simulink model "Freq_SimpleC_mex_new"  (R2020a)
settings: Solver=VariableStepAuto  StartTime=0.0  StopTime=50  FixedStep=0.02  MaxStep=1e-3  RelTol=1e-3
InitFcn:
  | M = 4; D = 1.5/100; Rp = 0.05; Tg = 0.2; Ki = 1.8;
libraries: commchan3 x1
settings Model: Creator=Niranjan.Bhujel  LastModifiedBy=astha.rai

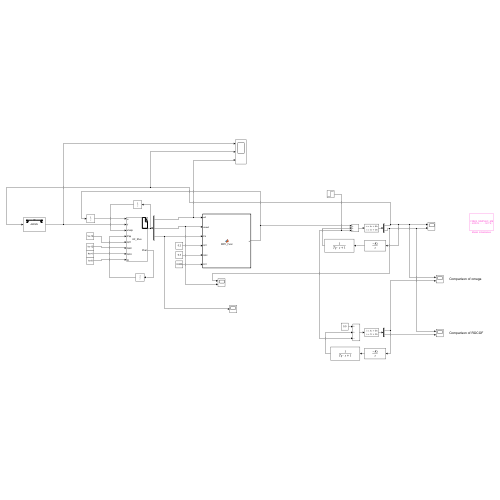
[thumbnail: Simulink's stored preview of the top-level diagram]
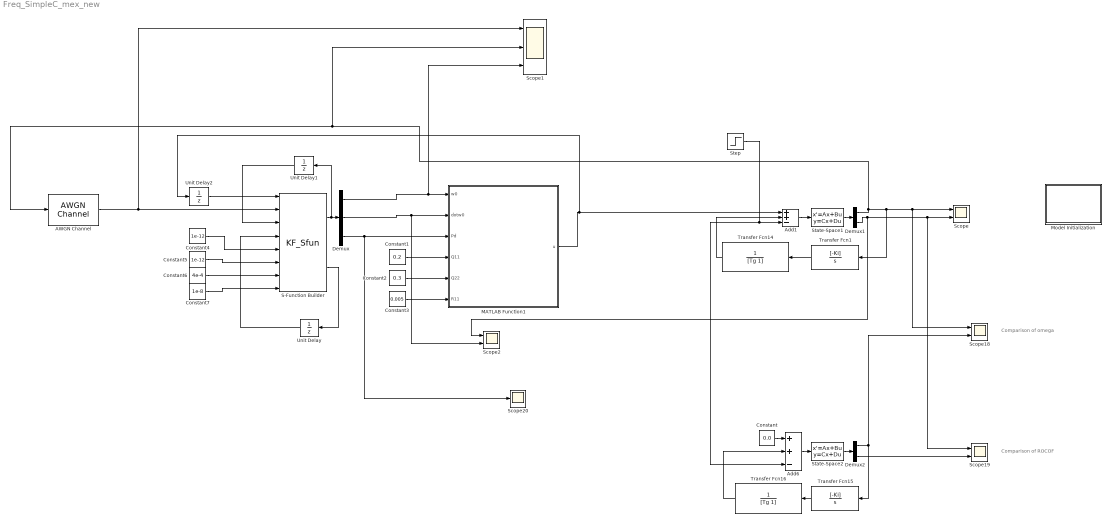
== system Freq_SimpleC_mex_new ==
  note: Comparison of omega
  note: Comparison of ROCOF
  AWGN Channel : commchan3/AWGN Channel  InputProcessing=Columns as channels (frame based)  seed=67  noiseMode=Variance from mask  EbNodB=10  EsNodB=10  SNRdB=10  bitsPerSym=1  Ps=1  Tsym=1  variance=1e-8
  Add1 : Sum  Inputs=++-
  Add6 : Sum  Inputs=++-
  Constant : Constant  Value=0.0
  Constant1 : Constant  Value=0.2
  Constant2 : Constant  Value=0.3
  Constant3 : Constant  Value=0.005
  Constant4 : Constant  Value=1e-12
  Constant5 : Constant  Value=1e-12
  Constant6 : Constant  Value=4e-4
  Constant7 : Constant  Value=1e-8
  Demux : Demux  Outputs=3
  Demux1 : Demux  Outputs=2
  Demux2 : Demux  Outputs=2
  MATLAB Function1 : MATLAB Function  TreatAsAtomicUnit=on  SystemSampleTime=0.02
      settings: MinAlgLoopOccurrences=on
  Model Initialization : Subsystem  mask(Model Functions){InitFcnX=M = 4; D = 1.5/100; Rp = 0.05; Tg = 0.2; Ki = 1.8;, prel=off, posl=off, inif=on, strf=off}
      mask prompts: InitFcnX "Initialisation"; prel "Preload Function"; posl "PostLoad Function"; inif "InitFcn"; strf "StartFcn"
      mask init:
      | currentBlock = gcb;
      | root = bdroot(currentBlock);
      | 
      | if ~strcmp(get_param(root,'BlockDiagramType'),'library')
      |     if prel==1
      |         set_param(root, 'PreLoadFcn', InitFcnX);
      |     else
      |         set_param(root, 'PreLoadFcn', '');
      |     end
      |     if inif==1
      |         set_param(root, 'InitFcn', InitFcnX);
      |     else
      |         set_param(root, 'InitFcn', '');
      |     end
      |     if strf==1
      |         set_param(root, 'StartFcn', InitFcnX);
      |     else
      |         set_param(root, 'StartFcn', '');
      |     end
      |     if posl==1
      |         set_param(root, 'PostLoadFcn', InitFcnX);
      |     else
      |         set_param(root, 'PostLoadFcn', '');
      |     end
      | end
      | 
      | pos = get_param(currentBlock, 'Position');
      | width = pos(3) - pos(1); height = pos(4) - pos(2);
      | txt = [ upper(root) '\n' '- InitFcn. . . . . '  get_param(root, 'InitFcn') ];
      settings: CopyFcn=set_param(gcb,'LinkStatus','inactive')
      mask Display: text(5, height*0.5, txt, 'horizontalAlignment', 'left', 'verticalAlignment', 'middle') ;
  S-Function Builder : S-Function  InitFcn=try, set_param(gcb,'FunctionName','KF_Sfun'), end  FunctionName=KF_Sfun  SFunctionModules=KF_Sfun_wrapper EKF_Func EKF_Func_Call  SFunctionDeploymentMode=off  EnableBusSupport=off  mask(S-Function Builder){}
      mask help: Simulink:masks:SFunctionBuilder_MD
      mask init:
      | val = [[.9  0.75 0.75 1 1 .9 .9 1]',[1 1 0.75 0.75 .9 .9 1 .9]'];try , sys = get_param(gcb,'SfunBuilderFcnName');if isempty(sys), sys = get_param(gcb,'FunctionName'); end,catch, sys = get_param(gcb,'FunctionName'); end
      settings: CopyFcn=set_param(gcbh,'LinkStatus','none')  PreSaveFcn=try, set_param(gcb,'FunctionName','KF_Sfun'), end  OpenFcn=sfunctionwizard(gcbh)
      mask Display:
      | plot(val(:,1),val(:,2))
      | disp(sys)
      | port_label('input',1,'u')
      | port_label('input',2,'y')
      | port_label('input',3,'xhatp')
      | port_label('input',4,'Pkp')
      | port_label('input',5,'Q11')
      | port_label('input',6,'Q22')
      | port_label('input',7,'Q33')
      | port_label('input',8,'R')
      | port_label('output',1,'xhat')
      | port_label('output',2,'Phat')
  Scope{,2,18..19} (4 alike) : Scope  NumInputPorts=2
  Scope1 : Scope  NumInputPorts=3
  Scope20 : Scope
  State-Space1 : StateSpace  A=[0 1;-(D/(M*Tg)+1/(Rp*M*Tg)) -(D/M + 1/Tg)]  B=[0;1/(M*Tg)]  C=eye(2)  D=zeros(2,1)  InitialCondition=0
  State-Space2 : StateSpace  A=[0 1;-(D/(M*Tg)+1/(Rp*M*Tg)) -(D/M + 1/Tg)]  B=[0;1/(M*Tg)]  C=eye(2)  D=zeros(2,1)  InitialCondition=0
  Step : Step  Time=10  After=0.75  SampleTime=0
  Transfer Fcn1 : TransferFcn  Numerator=[-Ki]  Denominator=[1 0]
  Transfer Fcn14 : TransferFcn  Denominator=[Tg 1]
  Transfer Fcn15 : TransferFcn  Numerator=[-Ki]  Denominator=[1 0]
  Transfer Fcn16 : TransferFcn  Denominator=[Tg 1]
  Unit Delay : UnitDelay  InitialCondition=1*diag([1, 1, 1])  SampleTime=0.02  HasFrameUpgradeWarning=on
  Unit Delay1 : UnitDelay  SampleTime=0.02  HasFrameUpgradeWarning=on
  Unit Delay2 : UnitDelay  SampleTime=0.02  HasFrameUpgradeWarning=on
  wires:
  Step/1 -> Add1/3, Add6/3
  Add1/1 -> State-Space1/1
  State-Space1/1 -> Demux1/1
  Transfer Fcn1/1 -> Transfer Fcn14/1
  Demux1/1 -> Transfer Fcn1/1, Scope18/1, Scope/1, Scope1/2, AWGN Channel/1
  Demux1/2 -> Scope2/1, Scope19/1, Scope/2
  Transfer Fcn15/1 -> Transfer Fcn16/1
  Add6/1 -> State-Space2/1
  Transfer Fcn16/1 -> Add6/2
  State-Space2/1 -> Demux2/1
  Demux2/1 -> Transfer Fcn15/1, Scope18/2
  Transfer Fcn14/1 -> Add1/2
  Demux2/2 -> Scope19/2
  MATLAB Function1/1(u) -> Unit Delay2/1, Add1/1
  Constant/1 -> Add6/1
  Constant1/1 -> MATLAB Function1/4(Q11)
  Constant2/1 -> MATLAB Function1/5(Q22)
  Constant3/1 -> MATLAB Function1/6(R11)
  Demux/3 -> Scope20/1, MATLAB Function1/3(Pd)
  S-Function Builder/1 -> Unit Delay1/1, Demux/1
  S-Function Builder/2 -> Unit Delay/1
  Unit Delay/1 -> S-Function Builder/4
  Unit Delay1/1 -> S-Function Builder/3
  Unit Delay2/1 -> S-Function Builder/1
  Constant4/1 -> S-Function Builder/5
  Constant5/1 -> S-Function Builder/6
  Constant6/1 -> S-Function Builder/7
  Constant7/1 -> S-Function Builder/8
  Demux/1 -> Scope1/3, MATLAB Function1/1(w0)
  Demux/2 -> Scope2/2, MATLAB Function1/2(dotw0)
  AWGN Channel/1 -> Scope1/1, S-Function Builder/2

== system Freq_SimpleC_mex_new/Model Initialization ==

== matlab function Freq_SimpleC_mex_new/MATLAB Function1 ==
  data: w0 input; u output; dotw0 input; Pd input; Q11 input; Q22 input; R11 input
function u = MPC_Func(w0, dotw0, Pd, Q11, Q22, R11)
% N = 50;
% Ts = 0.02;
coder.extrinsic('Mc');
u = 0.0;
u = Mc('M', w0, dotw0, Pd, Q11, Q22, R11);
